simulink model "Tarea_4_2"  (R2021a)
settings: Solver=VariableStepAuto  StartTime=0.0  StopTime=1000  RelTol=1e-3
values from neighbouring files (symbols this model uses):
  d = 0    [Tarea_4_v2.m]
  g = zeros(L,1)    [Tarea_4_v2.m]
  K = inv(G'*G + lambda*eye(M)) * G'    [Tarea_4_v2.m]
  M = 3    [Tarea_4_v2.m]
  N = 30    [Tarea_4_v2.m]
  P = 4    [Tarea_4_v2.m]
  sigma = 0.01    [Tarea_4_v2.m]
settings Model: Creator=Seb  LastModifiedBy=Seb

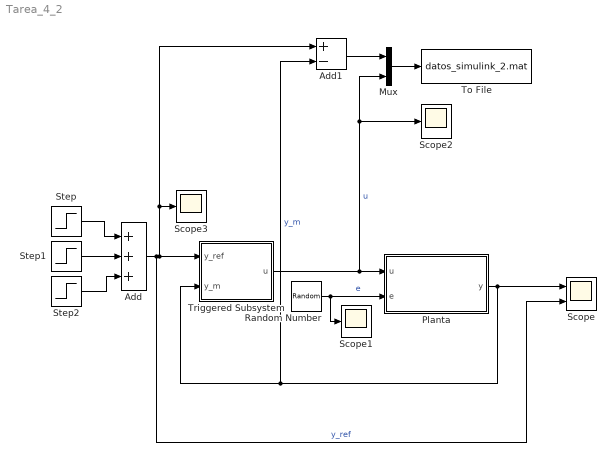
== system Tarea_4_2 ==
  Add : Sum  Inputs=+++
  Add1 : Sum  Inputs=+-
  Mux : Mux  Inputs=2
  Planta : Subsystem
  Random Number : RandomNumber  Variance=sigma^2  Seed=7  SampleTime=1
  Scope : Scope  NumInputPorts=2
  Scope1 : Scope
  Scope2 : Scope
  Scope3 : Scope
  Step : Step  Time=250  Before=1  After=2  SampleTime=0
  Step1 : Step  Time=500  After=2  SampleTime=0
  Step2 : Step  Time=750  After=-1  SampleTime=0
  To File : ToFile  Filename=datos_simulink_2.mat  MatrixName=datos  SampleTime=1
  Triggered Subsystem : Subsystem  TreatAsAtomicUnit=on
  wires:
  Random Number/1 -> Planta/2(e), Scope1/1  "e"
  Planta/1(y) -> Scope/1, Add1/2, Triggered Subsystem/2(y_m)  "y_m"
  Add/1 -> Scope/2, Add1/1, Scope3/1, Triggered Subsystem/1(y_ref)  "y_ref"
  Step/1 -> Add/1
  Step1/1 -> Add/2
  Step2/1 -> Add/3
  Triggered Subsystem/1(u) -> Scope2/1, Mux/2, Planta/1(u)  "u"
  Mux/1 -> To File/1
  Add1/1 -> Mux/1

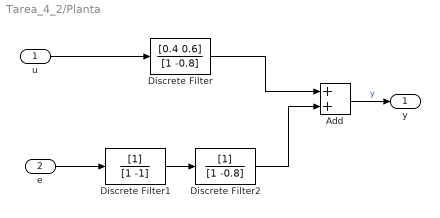
== system Tarea_4_2/Planta ==
  u : Inport
  e : Inport  Port=2
  Add : Sum
  Discrete Filter : DiscreteFilter  Numerator=[0.4 0.6]  Denominator=[1 -0.8]  SampleTime=1
  Discrete Filter1 : DiscreteFilter  Denominator=[1 -1]  SampleTime=1
  Discrete Filter2 : DiscreteFilter  Denominator=[1 -0.8]  SampleTime=1
  y : Outport
  wires:
  Add/1 -> y/1  "y"
  u/1 -> Discrete Filter/1
  Discrete Filter1/1 -> Discrete Filter2/1
  e/1 -> Discrete Filter1/1
  Discrete Filter/1 -> Add/1
  Discrete Filter2/1 -> Add/2

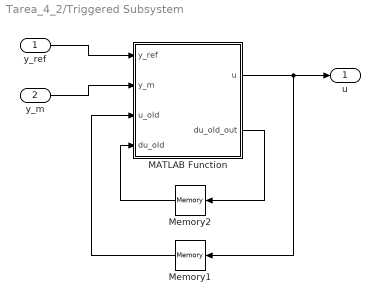
== system Tarea_4_2/Triggered Subsystem ==
  y_ref : Inport
  y_m : Inport  Port=2
  MATLAB Function : MATLAB Function  TreatAsAtomicUnit=on
  Memory1 : Memory  InheritSampleTime=on
  Memory2 : Memory  InitialCondition=zeros(30,1)  InheritSampleTime=on
  u : Outport
  wires:
  MATLAB Function/1(u) -> Memory1/1, u/1
  y_m/1 -> MATLAB Function/2(y_m)
  y_ref/1 -> MATLAB Function/1(y_ref)
  Memory1/1 -> MATLAB Function/3(u_old)
  Memory2/1 -> MATLAB Function/4(du_old)
  MATLAB Function/2(du_old_out) -> Memory2/1

== matlab function Tarea_4_2/Triggered Subsystem/MATLAB Function ==
  data: y_ref input; u output; y_m input; u_old input; du_old_out output size=30; du_old input; K parameter; P parameter; M parameter; g parameter; d parameter; N parameter
function [u,du_old_out] = DMC_fcn(y_ref, y_m, u_old, du_old, K, P, M, g, d, N)
% Función basada en la desarrollada por ayudante Francisco Rubio

f = zeros(P,1);

for k=(1:P)
    suma = 0;
    for i=(1:M)
        suma = suma + (g(k+i+d) - g(i+d))*du_old(i);
    end
    f(k) = y_m + suma;
end

du_act = K*(y_ref*ones(P,1)-f);
u = u_old + du_act(1);

du_old_out = zeros(30,1);
du_old_out(1) = du_act(1);
for i=(2:N-1)
    du_old_out(i) = du_old(i-1);
end

% du_old_out = [du_act(1); du_old(1:N-1)];
end
